simulink model "Flexy_tube_deltaU"  (R2020b)
settings: Solver=FixedStepAuto  StartTime=0.0  StopTime=15  FixedStep=Ts  RelTol=1e-3
values from neighbouring files (symbols this model uses):
  Ts = 0.01    [tube10.mat]    (also in tube13.mat; tube14.mat; tube16.mat; tube17.mat)
  us = 40    [tube10.mat]    (also in tube13.mat; tube14.mat; tube16.mat; tube17.mat)
  ys = 68    [tube10.mat]    (also in tube13.mat; tube14.mat; tube16.mat; tube17.mat)
undefined symbols (not defined in the file or in its folder): tube_eMPC_deltaU
libraries: flexy2_lib x2
settings Model: Creator=Michaela  LastModifiedBy=lgalc
settings SFSimCC: CustomCodeUndefinedFunction=UseInterfaceOnly

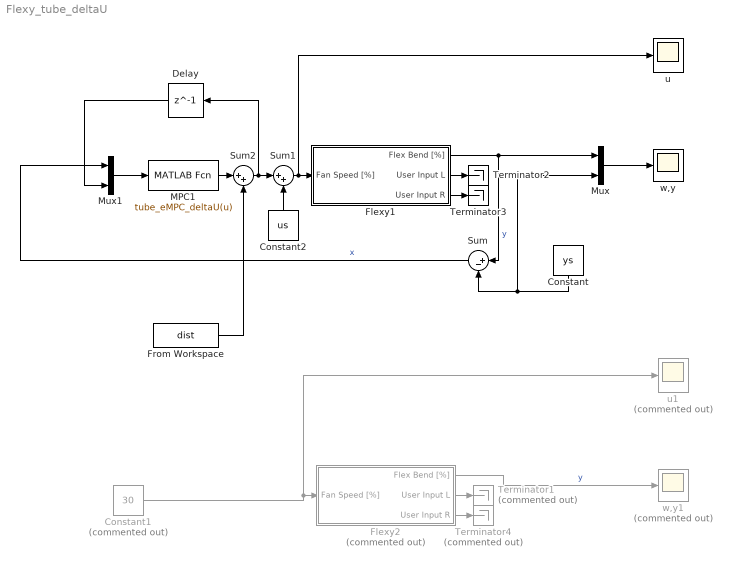
== system Flexy_tube_deltaU ==
  Constant : Constant  Value=ys
  Constant1 : Constant  Commented=on  Value=30
  Constant2 : Constant  Value=us
  Delay : Delay  DelayLength=1  InitialCondition=0-us
  Flexy1 : Subsystem
  Flexy2 : Subsystem  Commented=on
  From Workspace : FromWorkspace  VariableName=dist  OutDataTypeStr=double  SampleTime=-1
  MPC1 : MATLABFcn  MATLABFcn=tube_eMPC_deltaU(u)  SampleTime=Ts
  Mux : Mux  Inputs=2
  Mux1 : Mux  Inputs=2
  Sum : Sum  Inputs=|+-
  Sum1 : Sum  Inputs=|++
  Sum2 : Sum  Inputs=|++
  Terminator1 : Terminator  Commented=on
  Terminator2 : Terminator
  Terminator3 : Terminator
  Terminator4 : Terminator  Commented=on
  u : Scope
  u1 : Scope  Commented=on
  w,y : Scope
  w,y1 : Scope  Commented=on
  wires:
  Constant/1 -> Mux/2, Sum/2
  Flexy1/2(User Input L) -> Terminator2/1
  Flexy1/3(User Input R) -> Terminator3/1
  Flexy1/1(Flex Bend [%]) -> Mux/1, Sum/1  "y"
  Sum/1 -> Mux1/1  "x"
  MPC1/1 -> Sum2/1
  Constant1/1 -> Flexy2/1(Fan Speed [%]), u1/1
  Flexy2/1(Flex Bend [%]) -> w,y1/1  "y"
  Flexy2/2(User Input L) -> Terminator1/1
  Flexy2/3(User Input R) -> Terminator4/1
  Mux/1 -> w,y/1
  Mux1/1 -> MPC1/1
  Delay/1 -> Mux1/2
  Sum1/1 -> u/1, Flexy1/1(Fan Speed [%])
  Constant2/1 -> Sum1/2
  From Workspace/1 -> Sum2/2
  Sum2/1 -> Delay/1, Sum1/1

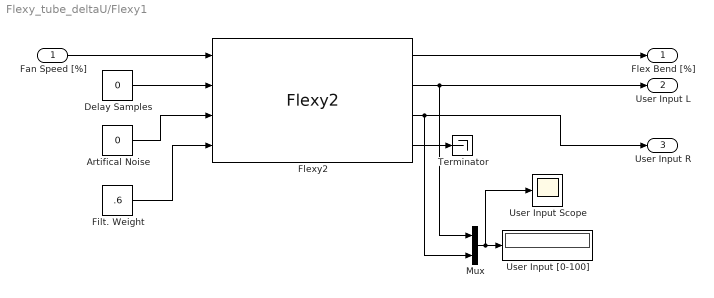
== system Flexy_tube_deltaU/Flexy1 ==
  Fan Speed [%] : Inport
  Artifical Noise : Constant  Value=0
  Delay Samples : Constant  Value=0
  Filt. Weight : Constant  Value=.6
  Flexy2 : flexy2_lib/Flexy2  SystemSampleTime=-1  VariantActivationTime=update diagram  Latency=0  AutoFrameSizeCalculation=off
  Mux : Mux  Inputs=2
  Terminator : Terminator
  User Input Scope : Scope
  User Input [0-100] : Display
  Flex Bend [%] : Outport
  User Input L : Outport  Port=2
  User Input R : Outport  Port=3
  wires:
  Fan Speed [%]/1 -> Flexy2/1
  Delay Samples/1 -> Flexy2/2
  Flexy2/2 -> Mux/1, User Input L/1
  Filt. Weight/1 -> Flexy2/4
  Flexy2/1 -> Flex Bend [%]/1
  Mux/1 -> User Input Scope/1, User Input [0-100]/1
  Flexy2/4 -> Terminator/1
  Flexy2/3 -> Mux/2, User Input R/1
  Artifical Noise/1 -> Flexy2/3

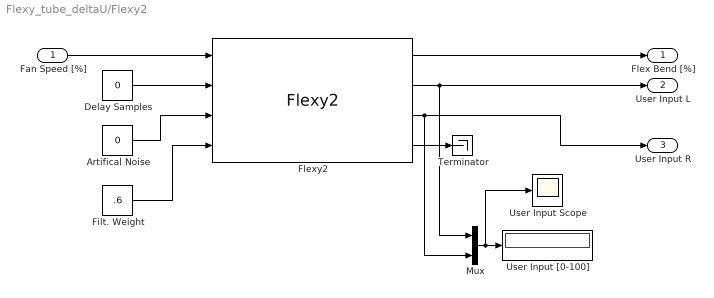
== system Flexy_tube_deltaU/Flexy2 ==
  Fan Speed [%] : Inport
  Artifical Noise : Constant  Value=0
  Delay Samples : Constant  Value=0
  Filt. Weight : Constant  Value=.6
  Flexy2 : flexy2_lib/Flexy2  SystemSampleTime=-1  VariantActivationTime=update diagram  Latency=0  AutoFrameSizeCalculation=off
  Mux : Mux  Inputs=2
  Terminator : Terminator
  User Input Scope : Scope
  User Input [0-100] : Display
  Flex Bend [%] : Outport
  User Input L : Outport  Port=2
  User Input R : Outport  Port=3
  wires:
  Fan Speed [%]/1 -> Flexy2/1
  Delay Samples/1 -> Flexy2/2
  Flexy2/2 -> Mux/1, User Input L/1
  Filt. Weight/1 -> Flexy2/4
  Flexy2/1 -> Flex Bend [%]/1
  Mux/1 -> User Input Scope/1, User Input [0-100]/1
  Flexy2/4 -> Terminator/1
  Flexy2/3 -> Mux/2, User Input R/1
  Artifical Noise/1 -> Flexy2/3
